simulink model "controller_experiment"  (R2023b)
settings: Solver=VariableStepAuto  StartTime=0.0  StopTime=7  RelTol=1e-3
values from neighbouring files (symbols this model uses):
  A = [Aaa Aab; Aba Abb]    [compensated_controller.m]    (also in controller_calc.m; driver_linearity.m = (ssx.*sy-sx.*sxy)/delta; observability_controllability.m = [0 1; 0 -(Bm/J+Km^2/(J*R))]; speed_profile.m = (ssx.*sy-sx.*sxy)/delta)
  AAd = [ ... (first row only)    [controller_calc.m]
  Adtilde = expm(Atilde*t_d)    [controller_calc.m]
  Aimp = [0 1; -Ke/Me -Be/Me]    [compensated_controller.m]    (also in controller_calc.m)
  B = [Bv Bt]    [compensated_controller.m]    (also in controller_calc.m; driver_linearity.m = (N.*sxy-sx.*sy)/delta; observability_controllability.m = [0 0; Km/(J*R) 1/J]; pwm_response_with_model.m = 2.7e-07)
  Bdtilde = Atilde\(Adtilde-1)*Btilde    [controller_calc.m]
  Bimp = [0 0; Ke/Me 1/Me]    [compensated_controller.m]    (also in controller_calc.m)
  Cdtilde = Ctilde    [controller_calc.m]
  Cimp = eye(2)    [compensated_controller.m]    (also in controller_calc.m)
  Ddtilde = Dtilde    [controller_calc.m]
  Dimp = zeros(2)    [compensated_controller.m]    (also in controller_calc.m)
  ei = 0    [controller_experiment_plot.m]
  nutildei = nui - ei    [controller_experiment_plot.m]
  t_d = 0.005    [motor_params.m]
  xi = [0; 0]    [controller_experiment_plot.m]    (also in stab_discrete.m = [0 0 0 x0 0 0]')
settings Model: Creator=tamas  LastModifiedBy=tamas

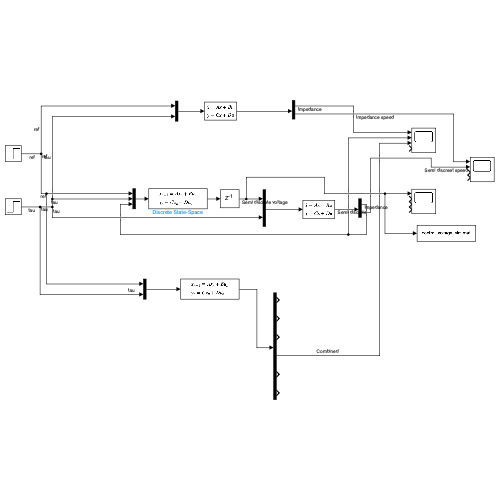
[thumbnail: Simulink's stored preview of the top-level diagram]
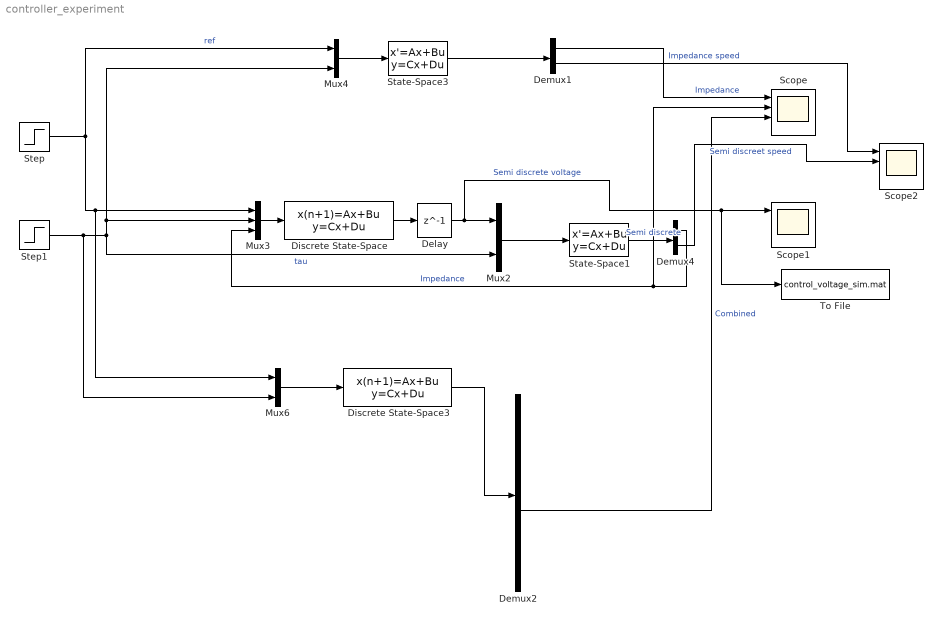
== system controller_experiment ==
  Delay : Delay  DelayLength=1  InitialCondition=0
  Demux1 : Demux  Outputs=2
  Demux2 : Demux  Outputs=6
  Demux4 : Demux  Outputs=2
  Discrete State-Space : DiscreteStateSpace  A=Adtilde  B=Bdtilde  C=Cdtilde  D=Ddtilde  InitialCondition=nutildei  SampleTime=t_d
  Discrete State-Space3 : DiscreteStateSpace  A=AAd  B=zeros([6, 2])  C=eye(6)  D=zeros([6, 2])  InitialCondition=[zeros(3, 1); xi; ei]  SampleTime=t_d
  Mux2 : Mux  Inputs=2
  Mux3 : Mux  Inputs=3
  Mux4 : Mux  Inputs=2
  Mux6 : Mux  Inputs=2
  Scope : Scope  NumInputPorts=4
  Scope1 : Scope  NumInputPorts=4
  Scope2 : Scope  NumInputPorts=4
  State-Space1 : StateSpace  A=A  B=B  C=eye(2)  D=zeros(2)  InitialCondition=xi
  State-Space3 : StateSpace  A=Aimp  B=Bimp  C=Cimp  D=Dimp  InitialCondition=xi
  Step : Step  Time=0  After=2.99*4.4  SampleTime=0
  Step1 : Step  Time=0  After=0  SampleTime=0
  To File : ToFile  Filename=control_voltage_sim.mat  MatrixName=control_voltage_sim  SaveFormat=Timeseries
  wires:
  State-Space3/1 -> Demux1/1
  Demux1/1 -> Scope/1  "Impedance"
  Mux4/1 -> State-Space3/1
  Mux2/1 -> State-Space1/1
  Delay/1 -> To File/1, Scope1/1, Mux2/1  "Semi discrete voltage"
  Mux3/1 -> Discrete State-Space/1
  Discrete State-Space/1 -> Delay/1
  Demux2/4 -> Scope/3  "Combined"
  Mux6/1 -> Discrete State-Space3/1
  Discrete State-Space3/1 -> Demux2/1
  Step1/1 -> Mux6/2, Mux2/2, Mux3/2, Mux4/2  "tau"
  Step/1 -> Mux6/1, Mux3/1, Mux4/1  "ref"
  Demux1/2 -> Scope2/1  "Impedance speed"
  State-Space1/1 -> Demux4/1  "Semi discrete"
  Demux4/2 -> Scope2/2  "Semi discreet speed"
  Demux4/1 -> Scope/2, Mux3/3  "Impedance"
